simulink model "lr_12"  (R2014b)
settings: Solver=ode45  StartTime=0.0  StopTime=50  MaxStep=0.001  RelTol=1e-3
settings Model: Creator=maksimka  LastModifiedBy=maksimka

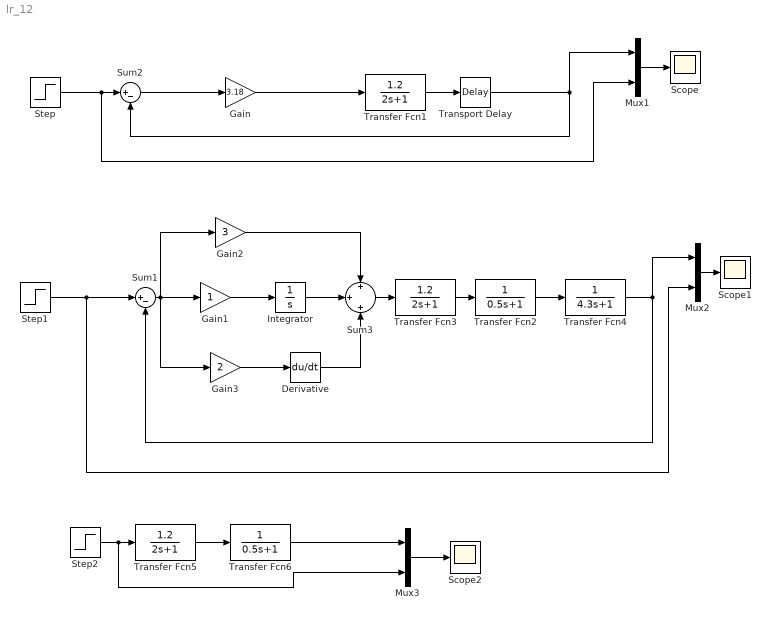
== system lr_12 ==
  Derivative : Derivative
  Gain : Gain  Gain=3.18
  Gain1 : Gain
  Gain2 : Gain  Gain=3
  Gain3 : Gain  Gain=2
  Integrator : Integrator
  Mux1 : Mux  Inputs=2
  Mux2 : Mux  Inputs=2
  Mux3 : Mux  Inputs=2
  Scope : Scope
      settings: TimeRange=20  YMin=-1  YMax=1  MaxDataPoints=50000
  Scope1 : Scope
      settings: TimeRange=20  YMin=-1  YMax=1  MaxDataPoints=50000
  Scope2 : Scope
      settings: TimeRange=20  YMin=-1  YMax=1  SaveName=ScopeData2  MaxDataPoints=50000
  Step : Step  SampleTime=0
  Step1 : Step  SampleTime=0
  Step2 : Step  SampleTime=0
  Sum1 : Sum  Inputs=|+-
  Sum2 : Sum  Inputs=|+-
  Sum3 : Sum  Inputs=+|+|+
  Transfer Fcn1 : TransferFcn  Numerator=[1.2]  Denominator=[2 1]
  Transfer Fcn2 : TransferFcn  Denominator=[0.5 1]
  Transfer Fcn3 : TransferFcn  Numerator=[1.2]  Denominator=[2 1]
  Transfer Fcn4 : TransferFcn  Denominator=[4.3 1]
  Transfer Fcn5 : TransferFcn  Numerator=[1.2]  Denominator=[2 1]
  Transfer Fcn6 : TransferFcn  Denominator=[0.5 1]
  Transport Delay : TransportDelay
  wires:
  Sum2/1 -> Gain/1
  Step/1 -> Mux1/2, Sum2/1
  Gain/1 -> Transfer Fcn1/1
  Mux1/1 -> Scope/1
  Transfer Fcn1/1 -> Transport Delay/1
  Transport Delay/1 -> Mux1/1, Sum2/2
  Sum1/1 -> Gain3/1, Gain1/1, Gain2/1
  Step1/1 -> Sum1/1, Mux2/2
  Gain1/1 -> Integrator/1
  Mux2/1 -> Scope1/1
  Integrator/1 -> Sum3/2
  Gain2/1 -> Sum3/1
  Gain3/1 -> Derivative/1
  Derivative/1 -> Sum3/3
  Sum3/1 -> Transfer Fcn3/1
  Transfer Fcn3/1 -> Transfer Fcn2/1
  Transfer Fcn2/1 -> Transfer Fcn4/1
  Transfer Fcn4/1 -> Sum1/2, Mux2/1
  Transfer Fcn5/1 -> Transfer Fcn6/1
  Transfer Fcn6/1 -> Mux3/1
  Step2/1 -> Mux3/2, Transfer Fcn5/1
  Mux3/1 -> Scope2/1
